simulink model "B_Modified_square_wave_Inverter"  (Simulink 10.1)
settings: Solver=ode3  StartTime=0.0  StopTime=inf  RelTol=1e-3  EnableMultiTasking=on
libraries: powerlib x10, simulink x3, powerlib_meascontrol x1
settings Model: Creator=ELECTRICAL-HOD  LastModifiedBy=Mateo C. Querol
settings DataIOCC: LimitDataPoints=on  SignalLoggingSaveFormat=ModelDataLogs
settings OptimizationCC: ExpressionDepthLimit=2147483647
settings DebuggingCC: SolverPrmCheckMsg=warning  FcnCallInpInsideContextMsg=warning  StateNameClashWarn=warning
settings ConfigComp: CovSFcnEnable=off
settings SimscapeCC: SimscapeNormalizeSystem=off

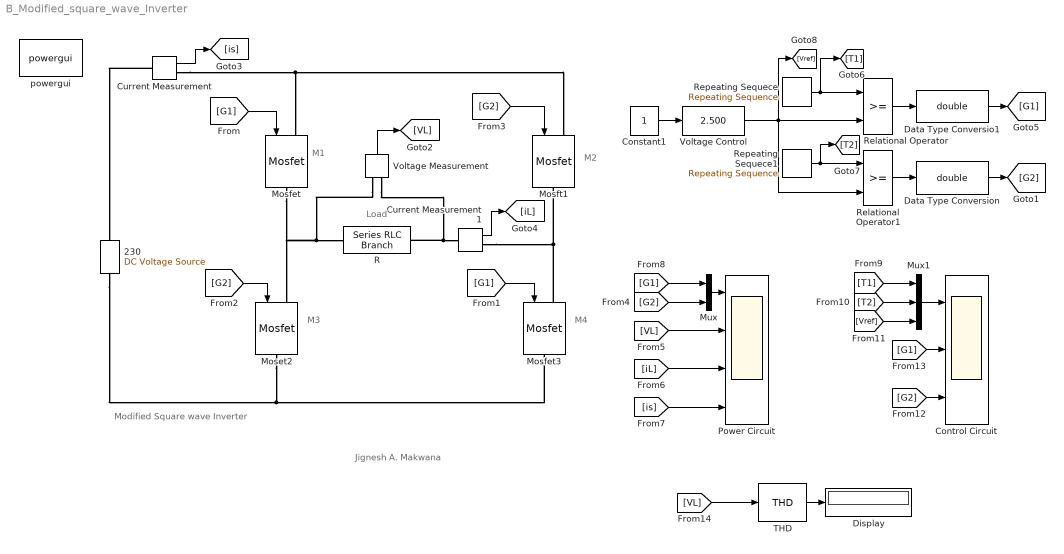
== system B_Modified_square_wave_Inverter ==
  note: Load
  note: M1
  note: M4
  note: M3
  note: M2
  note: Jignesh A. Makwana
  note: Modified Square wave Inverter
  230 : powerlib/Electrical Sources/DC Voltage Source  Amplitude=230  Measurements=None
  Constant1 : Constant
  Control Circuit : Scope  NumInputPorts=3
  Current Measurement : powerlib/Measurements/Current Measurement  PhasorSimulation=off  OutputType=Complex  PSBequivalent=0
  Current Measurement1 : powerlib/Measurements/Current Measurement  PhasorSimulation=off  OutputType=Complex  PSBequivalent=0
  Data Type Conversio1 : DataTypeConversion  OutDataTypeStr=double
  Data Type Conversion : DataTypeConversion  OutDataTypeStr=double
  Display : Display
  Moset2 : powerlib/Power Electronics/Mosfet  Ron=0.1  Lon=0  Rd=0.01  Vfd=0  IC=0  Rs=1e5  Cs=inf  Measurements=off
  Mosfet : powerlib/Power Electronics/Mosfet  Ron=0.1  Lon=0  Rd=0.01  Vfd=0  IC=0  Rs=1e5  Cs=inf  Measurements=off
  Mosfet3 : powerlib/Power Electronics/Mosfet  Ron=0.1  Lon=0  Rd=0.01  Vfd=0  IC=0  Rs=1e5  Cs=inf  Measurements=off
  Mosft1 : powerlib/Power Electronics/Mosfet  Ron=0.1  Lon=0  Rd=0.01  Vfd=0  IC=0  Rs=1e5  Cs=inf  Measurements=off
  Mux : Mux  Inputs=2
  Mux1 : Mux  Inputs=3
  Power Circuit : Scope  NumInputPorts=4
  R : powerlib/Elements/Series RLC Branch  LConnTagsString=__new0  RConnTagsString=__new0  BranchType=R  Resistance=1000  Inductance=15e-3  SetiL0=off  InitialCurrent=0  Capacitance=10e-6  Setx0=off  InitialVoltage=0  Measurements=None
  Relational Operator : RelationalOperator  OutDataTypeStr=boolean  RndMeth=Nearest
  Relational Operator1 : RelationalOperator  OutDataTypeStr=boolean  RndMeth=Nearest
  Repeating Sequece : simulink/Sources/Repeating Sequence  rep_seq_t=[0 0.01 0.02]  rep_seq_y=[-5.1 5.1 -5.1]
  Repeating Sequece1 : simulink/Sources/Repeating Sequence  rep_seq_t=[0 0.01 0.02]  rep_seq_y=[5.1 -5.1 5.1]
  THD : powerlib_meascontrol/Measurements/THD  Freq=50  Ts=0
  Voltage Control : simulink/Math Operations/Slider Gain  gain=2.500  low=0  high=5
  Voltage Measurement : powerlib/Measurements/Voltage Measurement  PhasorSimulation=off  OutputType=Complex  PSBequivalent=0
  powergui : powerlib/powergui  Priority=1  SimulationMode=Discrete  SampleTime=1e-6  frequency=60  Iterations=50  frequencyindice=0  Pbase=100e6  ErrMax=1e-4  UnitsV=kV  UnitsW=MW  buscounter=0  FunctionMessages=off  echomessages=off  EnableUseOfTLC=off  CurrentSourceSwitches=off  DisableSnubberDevices=off  DisableRonSwitches=off  DisableVfSwitches=off  DisplayEquations=off  AutomaticDiscreteSolvers=off  SolverType=Tustin  Interpol=off  ExternalGateDelay=off  methode=off  Ts=0  x0status=blocks  SPID=off  SwTol=0  HookPort=off  NonlinearTolerance=1e-4  nMaxIteration=100  ContinueOnMaxIteration=off  RestoreLinks=warning  ResistiveCurrentMeasurement=off  Frange=[0:2:500]  Ylog=off  Xlog=on  ShowGrid=off  save=off  variable=ZData  structure=0  ZoomFFT=off  StartTime=0.0  cycles=1  DisplayStyle=1  fundamental=60  FreqAxis=off  MaxFrequency=1000  frequencyindicesteady=1  RmsSteady=1  display=off
  wires:
  Voltage Measurement/1 -> [VL]
  Current Measurement/1 -> [is]
  Current Measurement1/1 -> [iL]
  [VL] -> Power Circuit/2
  [iL] -> Power Circuit/3
  [is] -> Power Circuit/4
  [G2] -> Mux/2
  [G1] -> Mux/1
  Mux/1 -> Power Circuit/1
  Repeating Sequece/1 -> Relational Operator/1, [T1]
  Voltage Control/1 -> Relational Operator/2, [Vref], Relational Operator1/2
  Repeating Sequece1/1 -> Relational Operator1/1, [T2]
  [G1] -> Mosfet3/1
  Relational Operator1/1 -> Data Type Conversion/1
  Relational Operator/1 -> Data Type Conversio1/1
  [G2] -> Mosft1/1
  [G2] -> Moset2/1
  [G1] -> Mosfet/1
  Data Type Conversion/1 -> [G2]
  Mux1/1 -> Control Circuit/1
  [T1] -> Mux1/1
  [T2] -> Mux1/2
  [Vref] -> Mux1/3
  [G1] -> Control Circuit/2
  [G2] -> Control Circuit/3
  Data Type Conversio1/1 -> [G1]
  Constant1/1 -> Voltage Control/1
  THD/1 -> Display/1
  [VL] -> THD/1
  connections:
  Mosfet/RConn1 -- Moset2/LConn1 -- Voltage Measurement/LConn1 -- R/LConn1
  Voltage Measurement/LConn2 -- R/RConn1 -- Current Measurement1/LConn1
  230/LConn1 -- Mosfet3/RConn1 -- Moset2/RConn1
  Current Measurement/RConn1 -- Mosft1/LConn1 -- Mosfet/LConn1
  Current Measurement/LConn1 -- 230/RConn1
  Mosfet3/LConn1 -- Mosft1/RConn1 -- Current Measurement1/RConn1
